simulink model "test18"  (R2021a)
settings: Solver=ode23tb  StartTime=0.0  StopTime=16  RelTol=1e-3
model workspace (MAT data in the model file):
  params = climate_p
  params.H = 7.99977069808
  params.A_f = 3100.00026794
  params.A_c = 3299.99999958
  params.minWindows = 0.49999998574
  params.alpha_i = 0.0143839885631
  params.cd_c = 8999.32112543
  params.T_ss = 285
values from neighbouring files (symbols this model uses):
  AR = 100    [test18_script.m]    (also in test18_ws.mat)
libraries: HORTISIM x4
settings Model: SimulationMode=accelerator  OrderedModelArguments=off  Creator=djoroya  LastModifiedBy=djoroya
settings DebuggingCC: UnconnectedInputMsg=none  UnconnectedOutputMsg=none  UnconnectedLineMsg=none

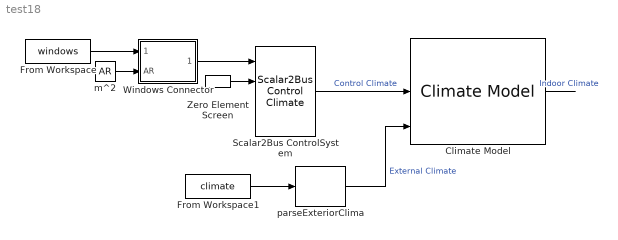
== system test18 ==
  Climate Model : HORTISIM/Climate/Models/Climate Model  params=climate_params  x0=cic
      settings: SourceProductName=Horti Simulator
  From Workspace : FromWorkspace  VariableName=windows
  From Workspace1 : FromWorkspace  VariableName=climate
  Scalar2Bus ControlSystem : HORTISIM/Other  Functions/Scalar2Bus  Control Climate  SystemSampleTime=-1  VariantActivationTime=update diagram  Latency=0  AutoFrameSizeCalculation=off
      settings: SourceProductName=Horti Simulator
  Windows Connector : Subsystem
  Zero Element Screen : HORTISIM/Other  Functions/Zero Element Screen  SystemSampleTime=-1  VariantActivationTime=update diagram  Latency=0  AutoFrameSizeCalculation=off
      settings: SourceProductName=Horti Simulator
  m^2 : Constant  Value=AR
  "parseExteriorClima " : HORTISIM/Other  Functions/parseExteriorClima  SystemSampleTime=-1  VariantActivationTime=update diagram  Latency=0  AutoFrameSizeCalculation=off
      settings: SourceProductName=Horti Simulator
  wires:
  Windows Connector/1(Windows) -> Scalar2Bus ControlSystem/1
  m^2/1 -> Windows Connector/2(AR)
  From Workspace/1 -> Windows Connector/1(value)
  Zero Element Screen/1 -> Scalar2Bus ControlSystem/2
  Climate Model/1 -> ?  "Indoor Climate"
  Scalar2Bus ControlSystem/1 -> Climate Model/2  "Control Climate"
  From Workspace1/1 -> "parseExteriorClima "/1
  "parseExteriorClima "/1 -> Climate Model/3  "External Climate"

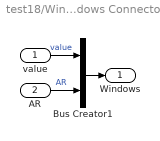
== system test18/Windows Connector ==
  value : Inport
  AR : Inport  Port=2
  Bus Creator1 : BusCreator  Inputs=2
  Windows : Outport
  wires:
  Bus Creator1/1 -> Windows/1
  value/1 -> Bus Creator1/1  "value"
  AR/1 -> Bus Creator1/2  "AR"
